simulink model "Phase_fullwave"  (R2017a)
settings: Solver=VariableStepDiscrete  StartTime=0.0  StopTime=.1  MaxStep=1e-4  RelTol=1e-3
libraries: powerlib x15
settings Model: Creator=asmit  LastModifiedBy=asmit

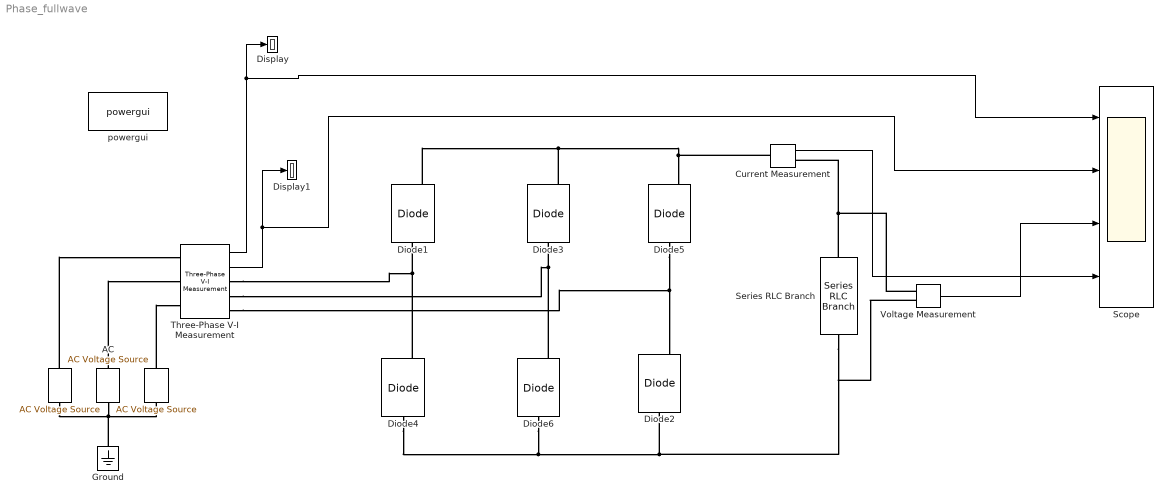
== system Phase_fullwave ==
  " " : powerlib/Electrical Sources/AC Voltage Source  Amplitude=100  Phase=0  Frequency=50  SampleTime=0  Measurements=None  BusType=swing  Pref=10e3  Qref=0  Qmin=-inf  Qmax=+inf
  " " : powerlib/Electrical Sources/AC Voltage Source  Amplitude=100  Phase=-240  Frequency=50  SampleTime=0  Measurements=None  BusType=swing  Pref=10e3  Qref=0  Qmin=-inf  Qmax=+inf
  "AC " : powerlib/Electrical Sources/AC Voltage Source  Amplitude=100  Phase=-120  Frequency=50  SampleTime=0  Measurements=None  BusType=swing  Pref=10e3  Qref=0  Qmin=-inf  Qmax=+inf
  Current Measurement : powerlib/Measurements/Current Measurement  PhasorSimulation=off  OutputType=Complex  PSBequivalent=0
  Diode{1..6} (6 alike) : powerlib/Power Electronics/Diode  Ron=0.001  Lon=0  Vf=0.8  IC=0  UseSnubber=0  Rs=500  Cs=250e-9  Measurements=on
  Display : Display
  Display1 : Display
  Ground : powerlib/Elements/Ground  LConnTagsString=a
  Scope : Scope  NumInputPorts=4
  Series RLC Branch : powerlib/Elements/Series RLC Branch  LConnTagsString=__new0  RConnTagsString=__new0  BranchType=R  Resistance=50  Inductance=1e-3  SetiL0=off  InitialCurrent=0  Capacitance=1e-6  Setx0=off  InitialVoltage=0  Measurements=None
  Three-Phase V-I Measurement : powerlib/Measurements/Three-Phase V-I Measurement  VoltageMeasurement=phase-to-ground  SetLabelV=off  LabelV=Vabc  Vpu=off  VpuLL=off  CurrentMeasurement=yes  SetLabelI=off  LabelI=Iabc  Ipu=off  Pbase=100e6  Vbase=500e3  OutputType=Complex  PhasorSimulation=off  PSBequivalent=0
  Voltage Measurement : powerlib/Measurements/Voltage Measurement  PhasorSimulation=off  OutputType=Complex  PSBequivalent=0
  powergui : powerlib/powergui  Priority=1  SimulationMode=Discrete  SampleTime=50e-6  frequency=60  Iterations=50  frequencyindice=50  Pbase=100e6  ErrMax=1e-4  UnitsV=kV  UnitsW=MW  buscounter=0  FunctionMessages=off  echomessages=off  EnableUseOfTLC=off  CurrentSourceSwitches=off  DisableSnubberDevices=off  DisableRonSwitches=off  DisableVfSwitches=off  DisplayEquations=off  SolverType=Tustin/Backward Euler (TBE)  Interpol=off  ExternalGateDelay=off  methode=off  Ts=100  x0status=blocks  SPID=on  SwTol=0  HookPort=off  RestoreLinks=warning  ResistiveCurrentMeasurement=off  Frange=[0:2:500]  Ylog=off  Xlog=on  ShowGrid=off  save=off  variable=ZData  structure=0  ZoomFFT=off  StartTime=0.0  cycles=1  DisplayStyle=1  fundamental=60  FreqAxis=off  MaxFrequency=1000  frequencyindicesteady=1  RmsSteady=1  display=off
  wires:
  Voltage Measurement/1 -> Scope/3
  Three-Phase V-I Measurement/1 -> Scope/1, Display/1
  Three-Phase V-I Measurement/2 -> Scope/2, Display1/1
  Current Measurement/1 -> Scope/4
  connections:
  " "/LConn1 -- Ground/LConn1 -- "AC "/LConn1
  Diode5/LConn1 -- Three-Phase V-I Measurement/RConn3 -- Diode2/RConn1
  Diode6/RConn1 -- Three-Phase V-I Measurement/RConn2 -- Diode3/LConn1
  Diode4/RConn1 -- Three-Phase V-I Measurement/RConn1 -- Diode1/LConn1
  Diode1/RConn1 -- Diode3/RConn1 -- Current Measurement/LConn1 -- Diode5/RConn1
  Diode4/LConn1 -- Diode6/LConn1 -- Voltage Measurement/LConn2 -- Series RLC Branch/RConn1 -- Diode2/LConn1
  " "/RConn1 -- Three-Phase V-I Measurement/LConn3
  "AC "/RConn1 -- Three-Phase V-I Measurement/LConn2
  " "/RConn1 -- Three-Phase V-I Measurement/LConn1
  Voltage Measurement/LConn1 -- Current Measurement/RConn1 -- Series RLC Branch/LConn1
